simulink model "ex_wavelets2"  (R2016b)
settings: Solver=FixedStepDiscrete  StartTime=0.0  StopTime=1024  FixedStep=1e-5  RelTol=1e-3  EnableMultiTasking=on
model workspace: external: MAT-File (data not in the file)
undefined symbols (not defined in the file or in its folder): ts
libraries: dspmlti4 x2
settings Model: ModifiedByFormat=The MathWorks Inc.  ExtModeTrigMode=oneshot  ExtModeArmWhenConnect=off  Creator=The MathWorks, Inc.  LastModifiedBy=The MathWorks Inc.
settings DataIOCC: SaveFormat=Array  SaveOutput=off  SaveTime=off  SignalLoggingName=sigsOut
settings OptimizationCC: BlockReduction=off  BooleanDataType=off  ExpressionDepthLimit=2147483647  InitFltsAndDblsToZero=on  EfficientMapNaN2IntZero=off  LifeSpan=inf
settings DebuggingCC: SaveWithParameterizedLinksMsg=none  UnderspecifiedInitializationDetection=Classic  MergeDetectMultiDrivingBlocksExec=none  SignalResolutionControl=TryResolveAllWithWarning  MultiTaskDSMMsg=warning  MultiTaskCondExecSysMsg=none  IntegerOverflowMsg=none  FcnCallInpInsideContextMsg=warning  StateNameClashWarn=warning  SFUnexpectedBacktrackingDiag=warning  SFNoUnconditionalDefaultTransitionDiag=warning  SFExecutionAtInitializationDiag=none  IntegerSaturationMsg=none
settings HardwareCC: ProdBitPerPointer=32  ProdBitPerSizeT=32  ProdBitPerPtrDiffT=32  ProdLargestAtomicFloat=None  ProdIntDivRoundTo=Undefined  ProdEndianess=Unspecified  ProdWordSize=32  ProdHWDeviceType=32-bit Generic  TargetUnknown=on
settings ModelReferenceCC: PropagateSignalLabelsOutOfModel=off
settings GRTTargetCC: TargetFcnLib=ansi_tfl_tmw.mat  TargetLangStandard=C89/C90 (ANSI)  GeneratePreprocessorConditionals=Disable all  CombineOutputUpdateFcns=off  GRTInterface=on
settings ConfigComp: CovMetricSettings=dw  CovHtmlReporting=on  CovSaveCumulativeToWorkspaceVar=on  CovSaveSingleToWorkspaceVar=on  CovExternalEMLEnable=off  CovSFcnEnable=off

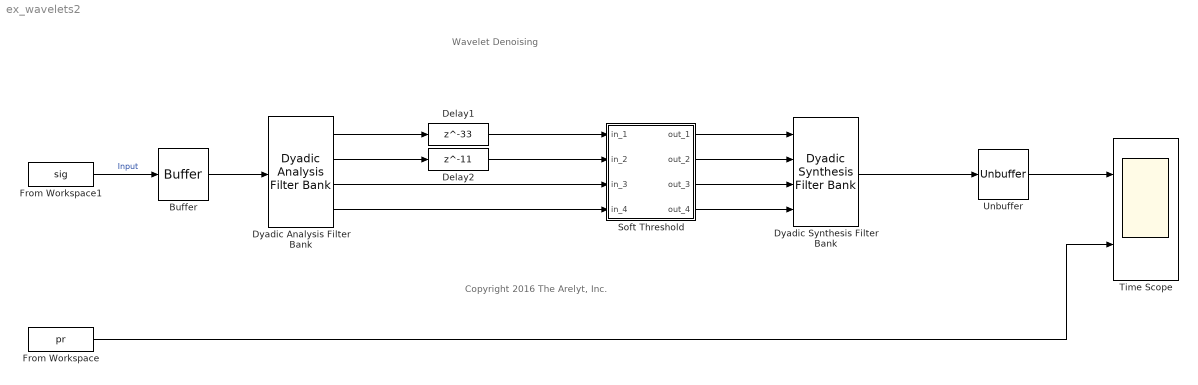
== system ex_wavelets2 ==
  note: Wavelet Denoising
  note: Copyright 2016 The Arelyt, Inc.
  Buffer : Buffer  N=32  TreatMby1Signals=One channel  OutputFrames=off
  Delay1 : Delay  DelayLength=33  InitialCondition=0  InputProcessing=Columns as channels (frame based)
  Delay2 : Delay  DelayLength=11  InitialCondition=0  InputProcessing=Columns as channels (frame based)
  Dyadic Analysis Filter Bank : dspmlti4/Dyadic Analysis Filter Bank  Wname=Biorthogonal  OrdRec_ordDec=[3 / 5]  Order=2  LPF=lod  HPF=hid  NumLevels=3  tree=Asymmetric  Output=Multiple ports  OutputFrames=off
  Dyadic Synthesis Filter Bank : dspmlti4/Dyadic Synthesis Filter Bank  Wname=Biorthogonal  OrdRec_ordDec=[3 / 5]  Order=2  LPF=lor  HPF=hir  NumLevels=3  tree=Asymmetric  Input=Multiple ports  OutputFrames=off
  From Workspace : FromWorkspace  VariableName=pr  SampleTime=ts
  From Workspace1 : FromWorkspace  VariableName=sig  SampleTime=ts
  Soft Threshold : Subsystem  mask(Soft Threshold){st=[3.694 2.803 1.411 0]}
      mask prompts: st "Vector of thresholds for each level:"
      mask help: Apply a soft threshold (deadzone transfer function) to each signal in the decomposition. First threshold applies to top-most filter bank output.
      mask init:
      | x=([-1 1 NaN 0 0 NaN -1 -.5 .5 1]+1)/2*.7+.15;
      | y=([0 0 NaN -1 1 NaN -1 0 0 1]+1)/2*.7+.05;
      mask Help: Vector of thresholds for each decomposition level.
      mask Display:
      | text(.1,.9,'Dead Zone')
      | plot(x,y)
  Time Scope : Scope  NumInputPorts=2
  Unbuffer : Unbuffer  SampleBasedProcessing=Same as frame based
  wires:
  Dyadic Analysis Filter Bank/1 -> Delay1/1
  Dyadic Analysis Filter Bank/2 -> Delay2/1
  Dyadic Analysis Filter Bank/4 -> Soft Threshold/4(in_4)
  Soft Threshold/4(out_4) -> Dyadic Synthesis Filter Bank/4
  Dyadic Analysis Filter Bank/3 -> Soft Threshold/3(in_3)
  Soft Threshold/3(out_3) -> Dyadic Synthesis Filter Bank/3
  Delay2/1 -> Soft Threshold/2(in_2)
  Soft Threshold/2(out_2) -> Dyadic Synthesis Filter Bank/2
  Delay1/1 -> Soft Threshold/1(in_1)
  Soft Threshold/1(out_1) -> Dyadic Synthesis Filter Bank/1
  Dyadic Synthesis Filter Bank/1 -> Unbuffer/1
  From Workspace/1 -> Time Scope/2
  Unbuffer/1 -> Time Scope/1
  Buffer/1 -> Dyadic Analysis Filter Bank/1
  From Workspace1/1 -> Buffer/1  "Input"

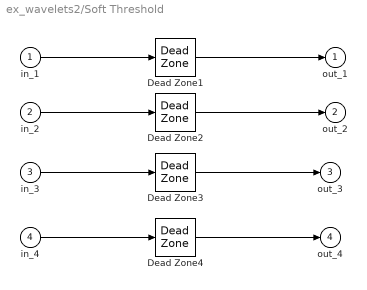
== system ex_wavelets2/Soft Threshold ==
  in_1 : Inport
  in_2 : Inport  Port=2
  in_3 : Inport  Port=3
  in_4 : Inport  Port=4
  Dead Zone1 : DeadZone  LowerValue=-st(1)  UpperValue=st(1)  ZeroCross=off  SaturateOnIntegerOverflow=on
  Dead Zone2 : DeadZone  LowerValue=-st(2)  UpperValue=st(2)  ZeroCross=off  SaturateOnIntegerOverflow=on
  Dead Zone3 : DeadZone  LowerValue=-st(3)  UpperValue=st(3)  ZeroCross=off  SaturateOnIntegerOverflow=on
  Dead Zone4 : DeadZone  LowerValue=-st(4)  UpperValue=st(4)  ZeroCross=off  SaturateOnIntegerOverflow=on
  out_1 : Outport
  out_2 : Outport  Port=2
  out_3 : Outport  Port=3
  out_4 : Outport  Port=4
  wires:
  in_1/1 -> Dead Zone1/1
  in_2/1 -> Dead Zone2/1
  in_3/1 -> Dead Zone3/1
  in_4/1 -> Dead Zone4/1
  Dead Zone1/1 -> out_1/1
  Dead Zone2/1 -> out_2/1
  Dead Zone3/1 -> out_3/1
  Dead Zone4/1 -> out_4/1
